simulink library "Decoders_Lib"  (Simulink 8.7)
settings: Solver=ode45  StartTime=0.0  StopTime=10.0  RelTol=1e-3
libraries: Computer_Library x17, commutil2 x5
(part 2 of 2)

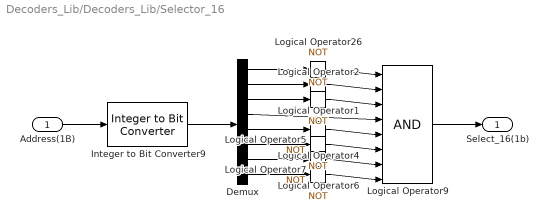
== system Decoders_Lib/Decoders_Lib/Selector_16 ==
  Address(1B) : Inport
  Demux : Demux  Outputs=8
  Integer to Bit Converter9 : commutil2/Integer to Bit Converter  nbits=8  signedInputValues=Unsigned  bitOrder=MSB first  outDtype=boolean
  Logical Operator{1..2,4..7,26} (7 alike) : Logic  Operator=NOT  Inputs=1  IconShape=distinctive  AllPortsSameDT=off  OutDataTypeStr=boolean
  Logical Operator9 : Logic  Inputs=8  IconShape=distinctive  AllPortsSameDT=off  OutDataTypeStr=boolean
  Select_16(1b) : Outport
  wires:
  Demux/8 -> Logical Operator7/1
  Logical Operator7/1 -> Logical Operator9/8
  Demux/7 -> Logical Operator6/1
  Logical Operator6/1 -> Logical Operator9/7
  Demux/6 -> Logical Operator5/1
  Logical Operator5/1 -> Logical Operator9/6
  Demux/5 -> Logical Operator4/1
  Logical Operator4/1 -> Logical Operator9/5
  Demux/4 -> Logical Operator9/4
  Demux/3 -> Logical Operator2/1
  Logical Operator2/1 -> Logical Operator9/3
  Demux/2 -> Logical Operator1/1
  Logical Operator1/1 -> Logical Operator9/2
  Logical Operator9/1 -> Select_16(1b)/1
  Demux/1 -> Logical Operator26/1
  Logical Operator26/1 -> Logical Operator9/1
  Address(1B)/1 -> Integer to Bit Converter9/1
  Integer to Bit Converter9/1 -> Demux/1

== system Decoders_Lib/Decoders_Lib/Selector_17 ==
  Address(1B) : Inport
  Bus Selector : BusSelector  OutputSignals=signal1,signal2,signal3,signal4,signal5,signal6,signal7,signal8
  Logical Operator{1..2,4..6,26} (6 alike) : Logic  Operator=NOT  Inputs=1  IconShape=distinctive  AllPortsSameDT=off  OutDataTypeStr=boolean
  Logical Operator9 : Logic  Inputs=8  IconShape=distinctive  AllPortsSameDT=off  OutDataTypeStr=boolean
  Select_17(1b) : Outport
  wires:
  Bus Selector/8 -> Logical Operator9/8  "<signal8>"
  Bus Selector/7 -> Logical Operator6/1  "<signal7>"
  Logical Operator6/1 -> Logical Operator9/7
  Bus Selector/6 -> Logical Operator5/1  "<signal6>"
  Logical Operator5/1 -> Logical Operator9/6
  Bus Selector/5 -> Logical Operator4/1  "<signal5>"
  Logical Operator4/1 -> Logical Operator9/5
  Bus Selector/4 -> Logical Operator9/4  "<signal4>"
  Bus Selector/3 -> Logical Operator2/1  "<signal3>"
  Logical Operator2/1 -> Logical Operator9/3
  Bus Selector/2 -> Logical Operator1/1  "<signal2>"
  Logical Operator1/1 -> Logical Operator9/2
  Logical Operator9/1 -> Select_17(1b)/1
  Bus Selector/1 -> Logical Operator26/1  "<signal1>"
  Logical Operator26/1 -> Logical Operator9/1
  Address(1B)/1 -> Bus Selector/1

== system Decoders_Lib/Decoders_Lib/Selector_18 ==
  Address(1B) : Inport
  Bus Selector : BusSelector  OutputSignals=signal1,signal2,signal3,signal4,signal5,signal6,signal7,signal8
  Logical Operator{1..2,4..5,7,26} (6 alike) : Logic  Operator=NOT  Inputs=1  IconShape=distinctive  AllPortsSameDT=off  OutDataTypeStr=boolean
  Logical Operator9 : Logic  Inputs=8  IconShape=distinctive  AllPortsSameDT=off  OutDataTypeStr=boolean
  Select_18(1b) : Outport
  wires:
  Bus Selector/8 -> Logical Operator7/1  "<signal8>"
  Logical Operator7/1 -> Logical Operator9/8
  Bus Selector/7 -> Logical Operator9/7  "<signal7>"
  Bus Selector/6 -> Logical Operator5/1  "<signal6>"
  Logical Operator5/1 -> Logical Operator9/6
  Bus Selector/5 -> Logical Operator4/1  "<signal5>"
  Logical Operator4/1 -> Logical Operator9/5
  Bus Selector/4 -> Logical Operator9/4  "<signal4>"
  Bus Selector/3 -> Logical Operator2/1  "<signal3>"
  Logical Operator2/1 -> Logical Operator9/3
  Bus Selector/2 -> Logical Operator1/1  "<signal2>"
  Logical Operator1/1 -> Logical Operator9/2
  Logical Operator9/1 -> Select_18(1b)/1
  Bus Selector/1 -> Logical Operator26/1  "<signal1>"
  Logical Operator26/1 -> Logical Operator9/1
  Address(1B)/1 -> Bus Selector/1

== system Decoders_Lib/Decoders_Lib/Selector_19 ==
  Address(1B) : Inport
  Demux : Demux  Outputs=8
  Integer to Bit Converter9 : commutil2/Integer to Bit Converter  nbits=8  signedInputValues=Unsigned  bitOrder=MSB first  outDtype=boolean
  Logical Operator{1..2,4..5,26} (5 alike) : Logic  Operator=NOT  Inputs=1  IconShape=distinctive  AllPortsSameDT=off  OutDataTypeStr=boolean
  Logical Operator9 : Logic  Inputs=8  IconShape=distinctive  AllPortsSameDT=off  OutDataTypeStr=boolean
  Select_19(1b) : Outport
  wires:
  Demux/8 -> Logical Operator9/8
  Demux/7 -> Logical Operator9/7
  Demux/6 -> Logical Operator5/1
  Logical Operator5/1 -> Logical Operator9/6
  Demux/5 -> Logical Operator4/1
  Logical Operator4/1 -> Logical Operator9/5
  Demux/4 -> Logical Operator9/4
  Demux/3 -> Logical Operator2/1
  Logical Operator2/1 -> Logical Operator9/3
  Demux/2 -> Logical Operator1/1
  Logical Operator1/1 -> Logical Operator9/2
  Logical Operator9/1 -> Select_19(1b)/1
  Demux/1 -> Logical Operator26/1
  Logical Operator26/1 -> Logical Operator9/1
  Address(1B)/1 -> Integer to Bit Converter9/1
  Integer to Bit Converter9/1 -> Demux/1

== system Decoders_Lib/Decoders_Lib/Selector_20 ==
  Address(1B) : Inport
  Bus Selector : BusSelector  OutputSignals=signal1,signal2,signal3,signal4,signal5,signal6,signal7,signal8
  Logical Operator{1..2,4,6..7,26} (6 alike) : Logic  Operator=NOT  Inputs=1  IconShape=distinctive  AllPortsSameDT=off  OutDataTypeStr=boolean
  Logical Operator9 : Logic  Inputs=8  IconShape=distinctive  AllPortsSameDT=off  OutDataTypeStr=boolean
  Select_20(1b) : Outport
  wires:
  Bus Selector/8 -> Logical Operator7/1  "<signal8>"
  Logical Operator7/1 -> Logical Operator9/8
  Bus Selector/7 -> Logical Operator6/1  "<signal7>"
  Logical Operator6/1 -> Logical Operator9/7
  Bus Selector/6 -> Logical Operator9/6  "<signal6>"
  Bus Selector/5 -> Logical Operator4/1  "<signal5>"
  Logical Operator4/1 -> Logical Operator9/5
  Bus Selector/4 -> Logical Operator9/4  "<signal4>"
  Bus Selector/3 -> Logical Operator2/1  "<signal3>"
  Logical Operator2/1 -> Logical Operator9/3
  Bus Selector/2 -> Logical Operator1/1  "<signal2>"
  Logical Operator1/1 -> Logical Operator9/2
  Logical Operator9/1 -> Select_20(1b)/1
  Bus Selector/1 -> Logical Operator26/1  "<signal1>"
  Logical Operator26/1 -> Logical Operator9/1
  Address(1B)/1 -> Bus Selector/1

== system Decoders_Lib/Decoders_Lib/Selector_21 ==
  Address(1B) : Inport
  Bus Selector : BusSelector  OutputSignals=signal1,signal2,signal3,signal4,signal5,signal6,signal7,signal8
  Logical Operator{1..2,4,6,26} (5 alike) : Logic  Operator=NOT  Inputs=1  IconShape=distinctive  AllPortsSameDT=off  OutDataTypeStr=boolean
  Logical Operator9 : Logic  Inputs=8  IconShape=distinctive  AllPortsSameDT=off  OutDataTypeStr=boolean
  Select_21(1b) : Outport
  wires:
  Bus Selector/8 -> Logical Operator9/8  "<signal8>"
  Bus Selector/7 -> Logical Operator6/1  "<signal7>"
  Logical Operator6/1 -> Logical Operator9/7
  Bus Selector/6 -> Logical Operator9/6  "<signal6>"
  Bus Selector/5 -> Logical Operator4/1  "<signal5>"
  Logical Operator4/1 -> Logical Operator9/5
  Bus Selector/4 -> Logical Operator9/4  "<signal4>"
  Bus Selector/3 -> Logical Operator2/1  "<signal3>"
  Logical Operator2/1 -> Logical Operator9/3
  Bus Selector/2 -> Logical Operator1/1  "<signal2>"
  Logical Operator1/1 -> Logical Operator9/2
  Logical Operator9/1 -> Select_21(1b)/1
  Bus Selector/1 -> Logical Operator26/1  "<signal1>"
  Logical Operator26/1 -> Logical Operator9/1
  Address(1B)/1 -> Bus Selector/1

== system Decoders_Lib/Decoders_Lib/Selector_22 ==
  Address(1B) : Inport
  Bus Selector : BusSelector  OutputSignals=signal1,signal2,signal3,signal4,signal5,signal6,signal7,signal8
  Logical Operator{1..2,4,7,26} (5 alike) : Logic  Operator=NOT  Inputs=1  IconShape=distinctive  AllPortsSameDT=off  OutDataTypeStr=boolean
  Logical Operator9 : Logic  Inputs=8  IconShape=distinctive  AllPortsSameDT=off  OutDataTypeStr=boolean
  Select_22(1b) : Outport
  wires:
  Bus Selector/8 -> Logical Operator7/1  "<signal8>"
  Logical Operator7/1 -> Logical Operator9/8
  Bus Selector/7 -> Logical Operator9/7  "<signal7>"
  Bus Selector/6 -> Logical Operator9/6  "<signal6>"
  Bus Selector/5 -> Logical Operator4/1  "<signal5>"
  Logical Operator4/1 -> Logical Operator9/5
  Bus Selector/4 -> Logical Operator9/4  "<signal4>"
  Bus Selector/3 -> Logical Operator2/1  "<signal3>"
  Logical Operator2/1 -> Logical Operator9/3
  Bus Selector/2 -> Logical Operator1/1  "<signal2>"
  Logical Operator1/1 -> Logical Operator9/2
  Logical Operator9/1 -> Select_22(1b)/1
  Bus Selector/1 -> Logical Operator26/1  "<signal1>"
  Logical Operator26/1 -> Logical Operator9/1
  Address(1B)/1 -> Bus Selector/1

== system Decoders_Lib/Decoders_Lib/Selector_23 ==
  Address(1B) : Inport
  Bus Selector : BusSelector  OutputSignals=signal1,signal2,signal3,signal4,signal5,signal6,signal7,signal8
  Logical Operator{1..2,4,26} (4 alike) : Logic  Operator=NOT  Inputs=1  IconShape=distinctive  AllPortsSameDT=off  OutDataTypeStr=boolean
  Logical Operator9 : Logic  Inputs=8  IconShape=distinctive  AllPortsSameDT=off  OutDataTypeStr=boolean
  Select_23(1b) : Outport
  wires:
  Bus Selector/8 -> Logical Operator9/8  "<signal8>"
  Bus Selector/7 -> Logical Operator9/7  "<signal7>"
  Bus Selector/6 -> Logical Operator9/6  "<signal6>"
  Bus Selector/5 -> Logical Operator4/1  "<signal5>"
  Logical Operator4/1 -> Logical Operator9/5
  Bus Selector/4 -> Logical Operator9/4  "<signal4>"
  Bus Selector/3 -> Logical Operator2/1  "<signal3>"
  Logical Operator2/1 -> Logical Operator9/3
  Bus Selector/2 -> Logical Operator1/1  "<signal2>"
  Logical Operator1/1 -> Logical Operator9/2
  Logical Operator9/1 -> Select_23(1b)/1
  Bus Selector/1 -> Logical Operator26/1  "<signal1>"
  Logical Operator26/1 -> Logical Operator9/1
  Address(1B)/1 -> Bus Selector/1

== system Decoders_Lib/Decoders_Lib/Selector_24 ==
  Address(1B) : Inport
  Bus Selector : BusSelector  OutputSignals=signal1,signal2,signal3,signal4,signal5,signal6,signal7,signal8
  Logical Operator{1..2,5..7,26} (6 alike) : Logic  Operator=NOT  Inputs=1  IconShape=distinctive  AllPortsSameDT=off  OutDataTypeStr=boolean
  Logical Operator9 : Logic  Inputs=8  IconShape=distinctive  AllPortsSameDT=off  OutDataTypeStr=boolean
  Select_24(1b) : Outport
  wires:
  Bus Selector/8 -> Logical Operator7/1  "<signal8>"
  Logical Operator7/1 -> Logical Operator9/8
  Bus Selector/7 -> Logical Operator6/1  "<signal7>"
  Logical Operator6/1 -> Logical Operator9/7
  Bus Selector/6 -> Logical Operator5/1  "<signal6>"
  Logical Operator5/1 -> Logical Operator9/6
  Bus Selector/5 -> Logical Operator9/5  "<signal5>"
  Bus Selector/4 -> Logical Operator9/4  "<signal4>"
  Bus Selector/3 -> Logical Operator2/1  "<signal3>"
  Logical Operator2/1 -> Logical Operator9/3
  Bus Selector/2 -> Logical Operator1/1  "<signal2>"
  Logical Operator1/1 -> Logical Operator9/2
  Logical Operator9/1 -> Select_24(1b)/1
  Bus Selector/1 -> Logical Operator26/1  "<signal1>"
  Logical Operator26/1 -> Logical Operator9/1
  Address(1B)/1 -> Bus Selector/1

== system Decoders_Lib/Decoders_Lib/Selector_25 ==
  Address(1B) : Inport
  Bus Selector : BusSelector  OutputSignals=signal1,signal2,signal3,signal4,signal5,signal6,signal7,signal8
  Logical Operator{1..2,5..6,26} (5 alike) : Logic  Operator=NOT  Inputs=1  IconShape=distinctive  AllPortsSameDT=off  OutDataTypeStr=boolean
  Logical Operator9 : Logic  Inputs=8  IconShape=distinctive  AllPortsSameDT=off  OutDataTypeStr=boolean
  Select_25(1b) : Outport
  wires:
  Bus Selector/8 -> Logical Operator9/8  "<signal8>"
  Bus Selector/7 -> Logical Operator6/1  "<signal7>"
  Logical Operator6/1 -> Logical Operator9/7
  Bus Selector/6 -> Logical Operator5/1  "<signal6>"
  Logical Operator5/1 -> Logical Operator9/6
  Bus Selector/5 -> Logical Operator9/5  "<signal5>"
  Bus Selector/4 -> Logical Operator9/4  "<signal4>"
  Bus Selector/3 -> Logical Operator2/1  "<signal3>"
  Logical Operator2/1 -> Logical Operator9/3
  Bus Selector/2 -> Logical Operator1/1  "<signal2>"
  Logical Operator1/1 -> Logical Operator9/2
  Logical Operator9/1 -> Select_25(1b)/1
  Bus Selector/1 -> Logical Operator26/1  "<signal1>"
  Logical Operator26/1 -> Logical Operator9/1
  Address(1B)/1 -> Bus Selector/1

== system Decoders_Lib/Decoders_Lib/Selector_26 ==
  Address(1B) : Inport
  Bus Selector : BusSelector  OutputSignals=signal1,signal2,signal3,signal4,signal5,signal6,signal7,signal8
  Logical Operator{1..2,5,7,26} (5 alike) : Logic  Operator=NOT  Inputs=1  IconShape=distinctive  AllPortsSameDT=off  OutDataTypeStr=boolean
  Logical Operator9 : Logic  Inputs=8  IconShape=distinctive  AllPortsSameDT=off  OutDataTypeStr=boolean
  Select_26(1b) : Outport
  wires:
  Bus Selector/8 -> Logical Operator7/1  "<signal8>"
  Logical Operator7/1 -> Logical Operator9/8
  Bus Selector/7 -> Logical Operator9/7  "<signal7>"
  Bus Selector/6 -> Logical Operator5/1  "<signal6>"
  Logical Operator5/1 -> Logical Operator9/6
  Bus Selector/5 -> Logical Operator9/5  "<signal5>"
  Bus Selector/4 -> Logical Operator9/4  "<signal4>"
  Bus Selector/3 -> Logical Operator2/1  "<signal3>"
  Logical Operator2/1 -> Logical Operator9/3
  Bus Selector/2 -> Logical Operator1/1  "<signal2>"
  Logical Operator1/1 -> Logical Operator9/2
  Logical Operator9/1 -> Select_26(1b)/1
  Bus Selector/1 -> Logical Operator26/1  "<signal1>"
  Logical Operator26/1 -> Logical Operator9/1
  Address(1B)/1 -> Bus Selector/1

== system Decoders_Lib/Decoders_Lib/Selector_27 ==
  Address(1B) : Inport
  Bus Selector : BusSelector  OutputSignals=signal1,signal2,signal3,signal4,signal5,signal6,signal7,signal8
  Logical Operator{1..2,5,26} (4 alike) : Logic  Operator=NOT  Inputs=1  IconShape=distinctive  AllPortsSameDT=off  OutDataTypeStr=boolean
  Logical Operator9 : Logic  Inputs=8  IconShape=distinctive  AllPortsSameDT=off  OutDataTypeStr=boolean
  Select_27(1b) : Outport
  wires:
  Bus Selector/8 -> Logical Operator9/8  "<signal8>"
  Bus Selector/7 -> Logical Operator9/7  "<signal7>"
  Bus Selector/6 -> Logical Operator5/1  "<signal6>"
  Logical Operator5/1 -> Logical Operator9/6
  Bus Selector/5 -> Logical Operator9/5  "<signal5>"
  Bus Selector/4 -> Logical Operator9/4  "<signal4>"
  Bus Selector/3 -> Logical Operator2/1  "<signal3>"
  Logical Operator2/1 -> Logical Operator9/3
  Bus Selector/2 -> Logical Operator1/1  "<signal2>"
  Logical Operator1/1 -> Logical Operator9/2
  Logical Operator9/1 -> Select_27(1b)/1
  Bus Selector/1 -> Logical Operator26/1  "<signal1>"
  Logical Operator26/1 -> Logical Operator9/1
  Address(1B)/1 -> Bus Selector/1

== system Decoders_Lib/Decoders_Lib/Selector_28 ==
  Address(1B) : Inport
  Bus Selector : BusSelector  OutputSignals=signal1,signal2,signal3,signal4,signal5,signal6,signal7,signal8
  Logical Operator{1..2,6..7,26} (5 alike) : Logic  Operator=NOT  Inputs=1  IconShape=distinctive  AllPortsSameDT=off  OutDataTypeStr=boolean
  Logical Operator9 : Logic  Inputs=8  IconShape=distinctive  AllPortsSameDT=off  OutDataTypeStr=boolean
  Select_28(1b) : Outport
  wires:
  Bus Selector/8 -> Logical Operator7/1  "<signal8>"
  Logical Operator7/1 -> Logical Operator9/8
  Bus Selector/7 -> Logical Operator6/1  "<signal7>"
  Logical Operator6/1 -> Logical Operator9/7
  Bus Selector/6 -> Logical Operator9/6  "<signal6>"
  Bus Selector/5 -> Logical Operator9/5  "<signal5>"
  Bus Selector/4 -> Logical Operator9/4  "<signal4>"
  Bus Selector/3 -> Logical Operator2/1  "<signal3>"
  Logical Operator2/1 -> Logical Operator9/3
  Bus Selector/2 -> Logical Operator1/1  "<signal2>"
  Logical Operator1/1 -> Logical Operator9/2
  Logical Operator9/1 -> Select_28(1b)/1
  Bus Selector/1 -> Logical Operator26/1  "<signal1>"
  Logical Operator26/1 -> Logical Operator9/1
  Address(1B)/1 -> Bus Selector/1

== system Decoders_Lib/Decoders_Lib/Selector_29 ==
  Address(1B) : Inport
  Bus Selector : BusSelector  OutputSignals=signal1,signal2,signal3,signal4,signal5,signal6,signal7,signal8
  Logical Operator{1..2,6,26} (4 alike) : Logic  Operator=NOT  Inputs=1  IconShape=distinctive  AllPortsSameDT=off  OutDataTypeStr=boolean
  Logical Operator9 : Logic  Inputs=8  IconShape=distinctive  AllPortsSameDT=off  OutDataTypeStr=boolean
  Select_29(1b) : Outport
  wires:
  Bus Selector/8 -> Logical Operator9/8  "<signal8>"
  Bus Selector/7 -> Logical Operator6/1  "<signal7>"
  Logical Operator6/1 -> Logical Operator9/7
  Bus Selector/6 -> Logical Operator9/6  "<signal6>"
  Bus Selector/5 -> Logical Operator9/5  "<signal5>"
  Bus Selector/4 -> Logical Operator9/4  "<signal4>"
  Bus Selector/3 -> Logical Operator2/1  "<signal3>"
  Logical Operator2/1 -> Logical Operator9/3
  Bus Selector/2 -> Logical Operator1/1  "<signal2>"
  Logical Operator1/1 -> Logical Operator9/2
  Logical Operator9/1 -> Select_29(1b)/1
  Bus Selector/1 -> Logical Operator26/1  "<signal1>"
  Logical Operator26/1 -> Logical Operator9/1
  Address(1B)/1 -> Bus Selector/1

== system Decoders_Lib/Decoders_Lib/Selector_30 ==
  Address(1B) : Inport
  Demux : Demux  Outputs=8
  Integer to Bit Converter9 : commutil2/Integer to Bit Converter  nbits=8  signedInputValues=Unsigned  bitOrder=MSB first  outDtype=boolean
  Logical Operator{1..2,7,26} (4 alike) : Logic  Operator=NOT  Inputs=1  IconShape=distinctive  AllPortsSameDT=off  OutDataTypeStr=boolean
  Logical Operator9 : Logic  Inputs=8  IconShape=distinctive  AllPortsSameDT=off  OutDataTypeStr=boolean
  Select_30(1b) : Outport
  wires:
  Demux/8 -> Logical Operator7/1
  Logical Operator7/1 -> Logical Operator9/8
  Demux/7 -> Logical Operator9/7
  Demux/6 -> Logical Operator9/6
  Demux/5 -> Logical Operator9/5
  Demux/4 -> Logical Operator9/4
  Demux/3 -> Logical Operator2/1
  Logical Operator2/1 -> Logical Operator9/3
  Demux/2 -> Logical Operator1/1
  Logical Operator1/1 -> Logical Operator9/2
  Logical Operator9/1 -> Select_30(1b)/1
  Demux/1 -> Logical Operator26/1
  Logical Operator26/1 -> Logical Operator9/1
  Address(1B)/1 -> Integer to Bit Converter9/1
  Integer to Bit Converter9/1 -> Demux/1

== system Decoders_Lib/Decoders_Lib/Selector_31 ==
  Address(1B) : Inport
  Demux : Demux  Outputs=8
  Integer to Bit Converter9 : commutil2/Integer to Bit Converter  nbits=8  signedInputValues=Unsigned  bitOrder=MSB first  outDtype=boolean
  Logical Operator1 : Logic  Operator=NOT  Inputs=1  IconShape=distinctive  AllPortsSameDT=off  OutDataTypeStr=boolean
  Logical Operator2 : Logic  Operator=NOT  Inputs=1  IconShape=distinctive  AllPortsSameDT=off  OutDataTypeStr=boolean
  Logical Operator26 : Logic  Operator=NOT  Inputs=1  IconShape=distinctive  AllPortsSameDT=off  OutDataTypeStr=boolean
  Logical Operator9 : Logic  Inputs=8  IconShape=distinctive  AllPortsSameDT=off  OutDataTypeStr=boolean
  Select_31(1b) : Outport
  wires:
  Demux/8 -> Logical Operator9/8
  Demux/7 -> Logical Operator9/7
  Demux/6 -> Logical Operator9/6
  Demux/5 -> Logical Operator9/5
  Demux/4 -> Logical Operator9/4
  Demux/3 -> Logical Operator2/1
  Logical Operator2/1 -> Logical Operator9/3
  Demux/2 -> Logical Operator1/1
  Logical Operator1/1 -> Logical Operator9/2
  Logical Operator9/1 -> Select_31(1b)/1
  Demux/1 -> Logical Operator26/1
  Logical Operator26/1 -> Logical Operator9/1
  Address(1B)/1 -> Integer to Bit Converter9/1
  Integer to Bit Converter9/1 -> Demux/1
